simulink model "model2d"  (Simulink 7.5)
settings: Solver=ode45  StartTime=0.0  StopTime=10.0  RelTol=1e-3
settings Model: Creator=aaron  LastModifiedBy=aaron
settings DebuggingCC: SolverPrmCheckMsg=none

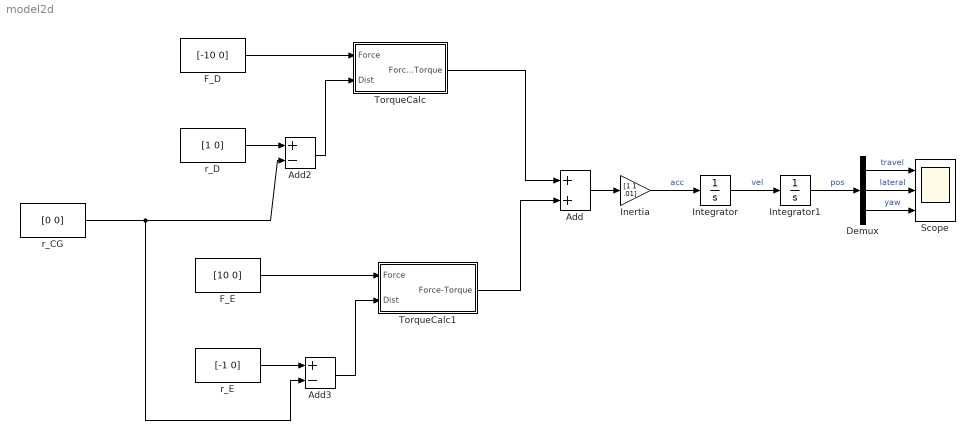
== system model2d ==
  Add : Sum  OutDataType=fixdt(1, 16)  OutScaling=2^-10
  Add2 : Sum  Inputs=+-  OutDataType=fixdt(1, 16)  OutScaling=2^-10
  Add3 : Sum  Inputs=+-  OutDataType=fixdt(1, 16)  OutScaling=2^-10
  Demux : Demux  Outputs=3
  F_D : Constant  Value=[-10 0]  OutDataType=fixdt(1, 16)  OutScaling=2^0
  F_E : Constant  Value=[10 0]  OutDataType=fixdt(1, 16)  OutScaling=2^0
  Inertia : Gain  Gain=[1 1 .01]  ParameterDataType=fixdt(1, 16)  ParameterScaling=2^0  OutDataType=fixdt(1, 16)  OutScaling=2^0
  Integrator : Integrator  InitialCondition=[100 0 0]
  Integrator1 : Integrator  InitialCondition=[0 0 0]
  Scope : Scope  NumInputPorts=3
      settings: YMin=-5~-5~-5  YMax=5~5~5  SaveName=position
  TorqueCalc : Subsystem
  TorqueCalc1 : Subsystem
  r_CG : Constant  Value=[0 0]  OutDataType=fixdt(1, 16)  OutScaling=2^0
  r_D : Constant  Value=[1 0]  OutDataType=fixdt(1, 16)  OutScaling=2^0
  r_E : Constant  Value=[-1 0]  OutDataType=fixdt(1, 16)  OutScaling=2^0
  wires:
  Integrator/1 -> Integrator1/1  "vel"
  F_D/1 -> TorqueCalc/1(Force)
  Inertia/1 -> Integrator/1  "acc"
  Add/1 -> Inertia/1
  TorqueCalc/1(Force-Torque) -> Add/1
  TorqueCalc1/1(Force-Torque) -> Add/2
  F_E/1 -> TorqueCalc1/1(Force)
  r_D/1 -> Add2/1
  r_CG/1 -> Add2/2, Add3/2
  r_E/1 -> Add3/1
  Add3/1 -> TorqueCalc1/2(Dist)
  Add2/1 -> TorqueCalc/2(Dist)
  Integrator1/1 -> Demux/1  "pos"
  Demux/1 -> Scope/1  "travel"
  Demux/2 -> Scope/2  "lateral"
  Demux/3 -> Scope/3  "yaw"

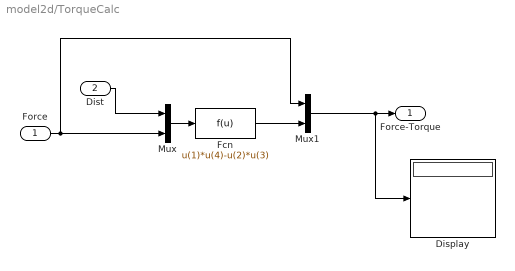
== system model2d/TorqueCalc ==
  Force : Inport
  Dist : Inport  Port=2
  Display : Display
  Fcn : Fcn  Expr=u(1)*u(4)-u(2)*u(3)
  Mux : Mux  Inputs=2
  Mux1 : Mux  Inputs=2
  Force-Torque : Outport
  wires:
  Force/1 -> Mux1/1, Mux/2
  Mux/1 -> Fcn/1
  Fcn/1 -> Mux1/2
  Mux1/1 -> Display/1, Force-Torque/1
  Dist/1 -> Mux/1

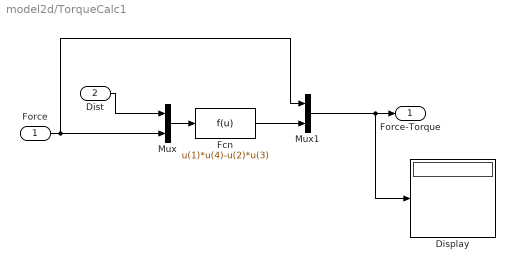
== system model2d/TorqueCalc1 ==
  Force : Inport
  Dist : Inport  Port=2
  Display : Display
  Fcn : Fcn  Expr=u(1)*u(4)-u(2)*u(3)
  Mux : Mux  Inputs=2
  Mux1 : Mux  Inputs=2
  Force-Torque : Outport
  wires:
  Force/1 -> Mux1/1, Mux/2
  Mux/1 -> Fcn/1
  Fcn/1 -> Mux1/2
  Mux1/1 -> Display/1, Force-Torque/1
  Dist/1 -> Mux/1
